simulink model "Prueba2_2016"  (R2016b)
settings: Solver=FixedStepAuto  StartTime=0.0  StopTime=10.0  RelTol=1e-3  EnableMultiTasking=on
undefined symbols (not defined in the file): Color, encod_L, encod_R, Gyro, Ultra
libraries: legoev3lib x14, simulink x1
settings Model: ExtModeTrigDuration=2  Creator=Nexel  LastModifiedBy=Nexel
settings SolverCC: PositivePriorityOrder=on
settings OptimizationCC: PassReuseOutputArgsThreshold=0  MaxStackSize=64
settings DebuggingCC: ParameterTunabilityLossMsg=error
settings HardwareCC: ProdBitPerPointer=32  ProdBitPerSizeT=32  ProdBitPerPtrDiffT=32  ProdLargestAtomicInteger=Long  ProdIntDivRoundTo=Floor  ProdWordSize=32  ProdHWDeviceType=ARM Compatible->ARM 9  UseEmbeddedCoderFeatures=off  UseSimulinkCoderFeatures=off
settings RTWCC: SystemTargetFile=ert.tlc  HardwareBoard=LEGO MINDSTORMS EV3  TLCOptions="-aInlineSetEventsForThisBaseRateFcn=TLC_FALSE -aSuppressMultiTaskScheduler=TLC_FALSE  -aRateBasedStepFcn=0"  TemplateMakefile=ert_default_tmf  Description=Embedded Coder  GenerateReport=on  Toolchain=Sourcery G++ Lite v2009q3  LaunchReport=on
settings CodeAppCC: ForceParamTrailComments=on  OperatorAnnotations=on
settings ERTTargetCC: MultiwordLength=256  ERTCustomFileBanners=off  SupportContinuousTime=on  SupportNonInlinedSFcns=on  RemoveResetFunc=off  SupportVariableSizeSignals=on  ModelStepFunctionPrototypeControlCompliant=off

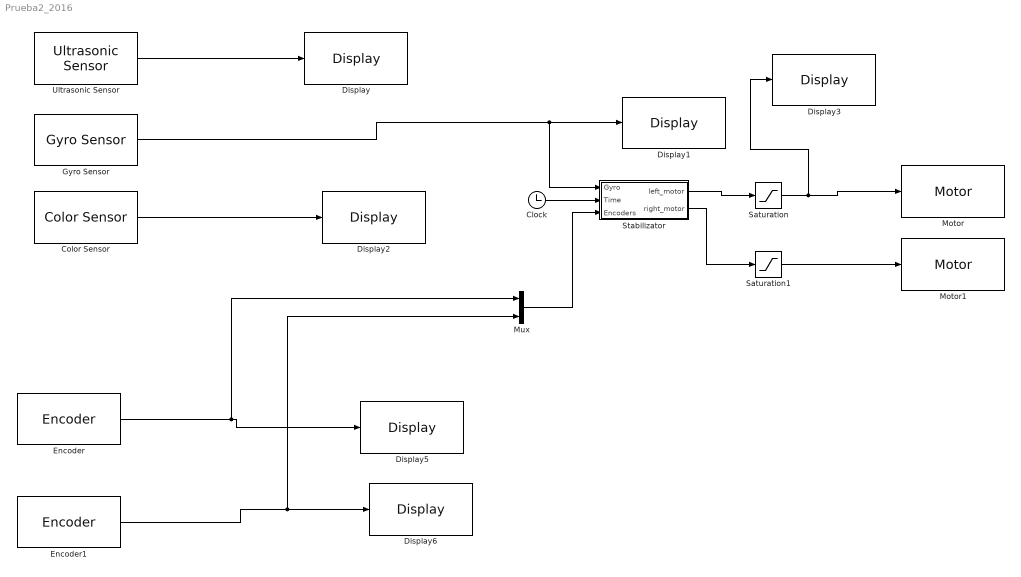
== system Prueba2_2016 ==
  Clock : Clock
      settings: Decimation=1000
  Color Sensor : legoev3lib/Color Sensor  portNumber=3  mode=Reflected light intensity  sampleTime=0.1
  Display : legoev3lib/Display  slcdStr=Ultra:  slcdLine=2  slcdFormat=Decimal
  Display1 : legoev3lib/Display  slcdStr=Gyro:  slcdLine=3  slcdFormat=Decimal
  Display2 : legoev3lib/Display  slcdStr=Color:  slcdLine=4  slcdFormat=Decimal
  Display3 : legoev3lib/Display  slcdStr=Left_mot  slcdLine=10  slcdFormat=Decimal
  Display5 : legoev3lib/Display  slcdStr=encod_L:  slcdLine=7  slcdFormat=Decimal
  Display6 : legoev3lib/Display  slcdStr=encod_R:  slcdLine=8  slcdFormat=Decimal
  Encoder : legoev3lib/Encoder  portNumber=C  opMode=No reset  sampleTime=0.1
  Encoder1 : legoev3lib/Encoder  portNumber=B  opMode=No reset  sampleTime=0.1
  Gyro Sensor : legoev3lib/Gyro Sensor  portNumber=2  sampleTime=0.1
  Motor : legoev3lib/Motor  sportNumber=C  sstopAction=Brake
  Motor1 : legoev3lib/Motor  sportNumber=B  sstopAction=Brake
  Mux : Mux  Inputs=2
  Saturation : Saturate  UpperLimit=20  LowerLimit=-20  LinearizeAsGain=off
  Saturation1 : Saturate  UpperLimit=20  LowerLimit=-20  LinearizeAsGain=off
  Stabilizator : Subsystem
  Ultrasonic Sensor : legoev3lib/Ultrasonic Sensor  PortNumber=4  sampleTime=0.1
  wires:
  Encoder/1 -> Mux/1, Display5/1
  Encoder1/1 -> Mux/2, Display6/1
  Color Sensor/1 -> Display2/1
  Gyro Sensor/1 -> Stabilizator/1("Gyro "), Display1/1
  Ultrasonic Sensor/1 -> Display/1
  Clock/1 -> Stabilizator/2(Time)
  Mux/1 -> Stabilizator/3("Encoders ")
  Saturation1/1 -> Motor1/1
  Saturation/1 -> Display3/1, Motor/1
  Stabilizator/1(left_motor) -> Saturation/1
  Stabilizator/2("right_motor ") -> Saturation1/1

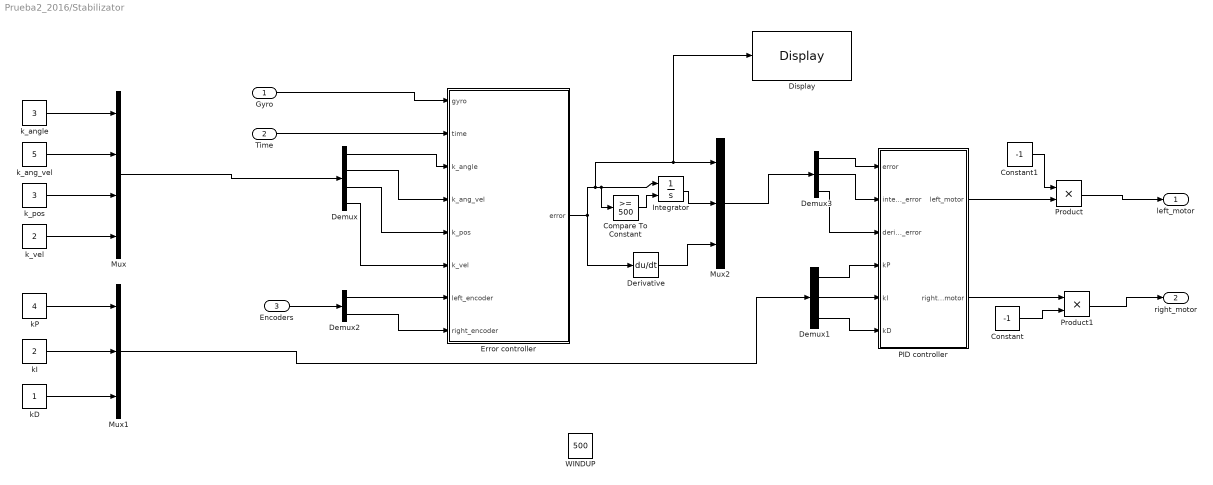
== system Prueba2_2016/Stabilizator ==
  "Gyro " : Inport
  Time : Inport  Port=2
  "Encoders " : Inport  Port=3
  Compare To Constant : simulink/Logic and Bit Operations/Compare To Constant  relop=>=  const=500  OutDataTypeStr=boolean
  Constant : Constant  Value=-1
  Constant1 : Constant  Value=-1
  Demux : Demux
  Demux1 : Demux  Outputs=3
  Demux2 : Demux  Outputs=2
  Demux3 : Demux  Outputs=3
  Derivative : Derivative
  Display : legoev3lib/Display  slcdStr=Error??  slcdLine=9  slcdFormat=Decimal
  Error controller : MATLAB Function  TreatAsAtomicUnit=on
  Integrator : Integrator  ExternalReset=rising  UpperSaturationLimit=500
  Mux : Mux
  Mux1 : Mux  Inputs=3
  Mux2 : Mux  Inputs=3
  "PID controller " : MATLAB Function  TreatAsAtomicUnit=on
  Product : Product
  Product1 : Product
  "WINDUP " : Constant  Value=500
  kD : Constant
  kI : Constant  Value=2
  kP : Constant  Value=4
  k_ang_vel : Constant  Value=5
  "k_angle " : Constant  Value=3
  k_pos : Constant  Value=3
  k_vel : Constant  Value=2
  left_motor : Outport
  "right_motor " : Outport  Port=2
  wires:
  "Gyro "/1 -> Error controller/1(gyro)
  "Encoders "/1 -> Demux2/1
  Demux1/1 -> "PID controller "/4(kP)
  Demux1/2 -> "PID controller "/5(kI)
  Demux1/3 -> "PID controller "/6(kD)
  Demux2/1 -> Error controller/7(left_encoder)
  Demux2/2 -> Error controller/8(right_encoder)
  Demux/1 -> Error controller/3(k_angle)
  Demux/2 -> Error controller/4(k_ang_vel)
  Demux/3 -> Error controller/5(k_pos)
  Demux/4 -> Error controller/6(k_vel)
  "k_angle "/1 -> Mux/1
  k_ang_vel/1 -> Mux/2
  k_pos/1 -> Mux/3
  k_vel/1 -> Mux/4
  Mux/1 -> Demux/1
  kP/1 -> Mux1/1
  kI/1 -> Mux1/2
  kD/1 -> Mux1/3
  Mux1/1 -> Demux1/1
  Time/1 -> Error controller/2(time)
  Error controller/1(error) -> Derivative/1, Display/1, Mux2/1, Compare To Constant/1, Integrator/1
  Integrator/1 -> Mux2/2
  Derivative/1 -> Mux2/3
  Demux3/2 -> "PID controller "/2(integral_error)
  Demux3/1 -> "PID controller "/1(error)
  Demux3/3 -> "PID controller "/3(derivative_error)
  Mux2/1 -> Demux3/1
  "PID controller "/1(left_motor) -> Product/2
  "PID controller "/2(right_motor) -> Product1/1
  Constant/1 -> Product1/2
  Product1/1 -> "right_motor "/1
  Constant1/1 -> Product/1
  Product/1 -> left_motor/1
  Compare To Constant/1 -> Integrator/2

== matlab function Prueba2_2016/Stabilizator/PID controller  ==
  data: error input; left_motor output; integral_error input; derivative_error input; right_motor output; kP input; kI input; kD input
function [left_motor, right_motor] = PID_controller(error, integral_error, derivative_error, kP,kI,kD)
%% Calculate output
    u = kP * error + kI * integral_error + kD * derivative_error;
    left_motor = int32(u); right_motor = int32(u);
end

== matlab function Prueba2_2016/Stabilizator/Error controller ==
  data: gyro input; error output; time input; k_angle input; k_ang_vel input; k_pos input; k_vel input; left_encoder input; right_encoder input
function error  = error_controller(gyro, time, k_angle, k_ang_vel, k_pos, k_vel, left_encoder, right_encoder)
    persistent prev_angle prev_pos_x prev_time rnd_min rnd_max
    if isempty(prev_angle)
        prev_angle = double(0);
        prev_pos_x = double(0);
        prev_time = double(0);
        rnd_min = -5;
        rnd_max = 5;
    end
    delayed_time = double(time) - prev_time;
    %% Calculate Angle
    angle = prev_angle + double(delayed_time) * -gyro;
    %% Calculate position
    pos_x = double((left_encoder + right_encoder) / 2);
    x_ref = pos_x + (rnd_min + rand * (rnd_max - rnd_min));
    %% Calculate deviation
    deviation = pos_x - x_ref;
    %% Calculate velocity
    velocity = double((pos_x - prev_pos_x)/delayed_time);
    %% Calculate error
    error = double(k_angle*double(angle) + k_ang_vel*double(-gyro) + k_pos * double(deviation) + k_vel * double(velocity));
    %% Update persistent
        prev_angle = double(angle);
        prev_pos_x = double(pos_x);
        prev_time = double(time);
end
